simulink library "cdsBit2Word"  (Simulink 7.1)
settings Model: Creator=Rolf  LastModifiedBy=maronsson

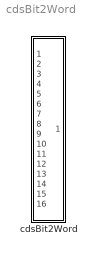
== system cdsBit2Word ==
  cdsBit2Word : Subsystem  Tag=cdsBit2Word  Description=Forms single 16 bit integer from 16 0/1 inputs.
      settings: AttributesFormatString=%<Tag>

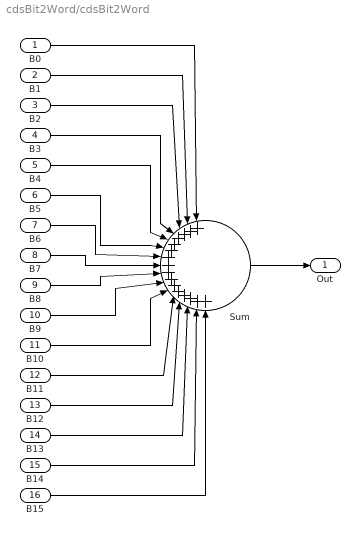
== system cdsBit2Word/cdsBit2Word ==
  B0 : Inport  OutDataType=sfix(16)  OutScaling=2^0
  B1 : Inport  Port=2  OutDataType=sfix(16)  OutScaling=2^0
  B2 : Inport  Port=3  OutDataType=sfix(16)  OutScaling=2^0
  B3 : Inport  Port=4  OutDataType=sfix(16)  OutScaling=2^0
  B4 : Inport  Port=5  OutDataType=sfix(16)  OutScaling=2^0
  B5 : Inport  Port=6  OutDataType=sfix(16)  OutScaling=2^0
  B6 : Inport  Port=7  OutDataType=sfix(16)  OutScaling=2^0
  B7 : Inport  Port=8  OutDataType=sfix(16)  OutScaling=2^0
  B8 : Inport  Port=9  OutDataType=sfix(16)  OutScaling=2^0
  B9 : Inport  Port=10  OutDataType=sfix(16)  OutScaling=2^0
  B10 : Inport  Port=11  OutDataType=sfix(16)  OutScaling=2^0
  B11 : Inport  Port=12  OutDataType=sfix(16)  OutScaling=2^0
  B12 : Inport  Port=13  OutDataType=sfix(16)  OutScaling=2^0
  B13 : Inport  Port=14  OutDataType=sfix(16)  OutScaling=2^0
  B14 : Inport  Port=15  OutDataType=sfix(16)  OutScaling=2^0
  B15 : Inport  Port=16  OutDataType=sfix(16)  OutScaling=2^0
  Sum : Sum  Inputs=|++++++++++++++++  OutDataType=sfix(16)  OutScaling=2^0
  Out : Outport  OutDataType=sfix(16)  OutScaling=2^0
  wires:
  B0/1 -> Sum/1
  B1/1 -> Sum/2
  B2/1 -> Sum/3
  B3/1 -> Sum/4
  B4/1 -> Sum/5
  B5/1 -> Sum/6
  B6/1 -> Sum/7
  B7/1 -> Sum/8
  B8/1 -> Sum/9
  B9/1 -> Sum/10
  B10/1 -> Sum/11
  B11/1 -> Sum/12
  B12/1 -> Sum/13
  B13/1 -> Sum/14
  B14/1 -> Sum/15
  B15/1 -> Sum/16
  Sum/1 -> Out/1
